simulink model "forhead"  (R2018a)
settings: Solver=FixedStepDiscrete  StartTime=0.0  StopTime=1  RelTol=1e-3
InitFcn:
  | mbd_pnt_consistency_checks(bdroot(gcs));
undefined symbols (not defined in the file): C11, P16
libraries: mbd_pnt_ec_toolbox x2
settings Model: Creator=oolonthegreat  LastModifiedBy=oolonthegreat
settings DataIOCC: ExternalInput=off  InitialState=off  SaveOutput=off  SignalLogging=off  SaveTime=off
settings OptimizationCC: DefaultParameterBehavior=Inlined  EnhancedBackFolding=on  PassReuseOutputArgsAs=Individual arguments  OptimizeBlockOrder=speed  DifferentSizesBufferReuse=on  OptimizationCustomize=off
settings DebuggingCC: InheritedTsInSrcMsg=none  SingleTaskRateTransMsg=error  ParameterTunabilityLossMsg=error  UnconnectedInputMsg=error  UnconnectedOutputMsg=error  UnconnectedLineMsg=error  UnknownTsInhSupMsg=error
settings HardwareCC: ProdBitPerPointer=32  ProdBitPerSizeT=32  ProdBitPerPtrDiffT=32  ProdLargestAtomicInteger=Long  ProdLargestAtomicFloat=Double  ProdEndianess=BigEndian  ProdWordSize=32  ProdHWDeviceType=Motorola PowerPC
settings SFSimCC: MATLABDynamicMemAlloc=off
settings RTWCC: SystemTargetFile=mbd_pnt.tlc  MakeCommand=mbd_pnt_make_rtw COPY_MDLREF_INCLUDES=0  TemplateMakefile=mbd_pnt.tmf  PostCodeGenCommand=mbd_pnt_analyzegencode(buildInfo)  Description=Model Based Design Toolbox MPC574xP Code Generation Target  GenerateReport=on  IncludeHyperlinkInReport=on  LaunchReport=on  GenerateTraceInfo=on  GenerateTraceReport=on  GenerateTraceReportSl=on  GenerateTraceReportSf=on  GenerateTraceReportEml=on
settings CodeAppCC: ForceParamTrailComments=on  IgnoreCustomStorageClasses=off  OperatorAnnotations=on  SimulinkDataObjDesc=on  SFDataObjDesc=on  InsertBlockDesc=on
settings STFCustomTargetCC: TargetLangStandard=C99 (ISO)  MultiwordLength=256  CombineOutputUpdateFcns=on  SuppressErrorStatus=on  ERTCustomFileBanners=on  SupportContinuousTime=off  SupportNonInlinedSFcns=off  RemoveResetFunc=on  MATLABClassNameForMDSCustomization=Simulink.SoftwareTarget.ERTCustomization  GRTInterface=off  SystemTargetFile=mbd_pnt.tlc
settings ERTTargetCC: TargetLangStandard=C99 (ISO)  ParMdlRefBuildCompliant=off  CompOptLevelCompliant=off  ConcurrentExecutionCompliant=off  SuppressErrorStatus=on  ModelStepFunctionPrototypeControlCompliant=off  CPPClassGenCompliant=off  UseToolchainInfoCompliant=off  InlinedParameterPlacement=NonHierarchical  ERTCustomFileTemplate=example_file_process.tlc

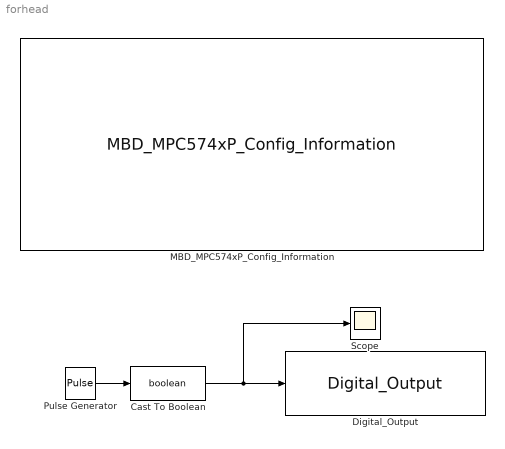
== system forhead ==
  Cast To Boolean : DataTypeConversion  OutDataTypeStr=boolean
  Digital_Output : mbd_pnt_ec_toolbox/MPC574xP/Peripheral Interface Blocks/Digital_Output  gpio_outputs="43   : C11 :  [80]   : [97]   : [P16]"  pinNum=[80]  pcrNum=43
      settings: SourceProductName=Model Based Design Toolbox for MPC574xP
  MBD_MPC574xP_Config_Information : mbd_pnt_ec_toolbox/MPC574xP/MBD_MPC574xP_Config_Information  disp_str=|  config_params=[]
      | System Clock : 200 MHz
      | Target : MPC5744P
      | Package : 144LQFP
      | XTAL Freq : 40 MHz
      | Compiler : S32 Design Studio
      | Target Type : FLASH
      | Global Interrupt Priority : 8
      | System Tick Interrupt Priority : 12
      | Freemaster : None;
      | Download Code after build : (COM5,115200)
      settings: SourceProductName=Model Based Design Toolbox for MPC574xP
  Pulse Generator : DiscretePulseGenerator  PulseType=Time based  Period=0.4492957746479  PulseWidth=40
  Scope : Scope
  wires:
  Pulse Generator/1 -> Cast To Boolean/1
  Cast To Boolean/1 -> Scope/1, Digital_Output/1
